simulink model "Simulation"  (R2024b)
settings: Solver=VariableStepAuto  StartTime=0.0  StopTime=10  RelTol=1e-3
model workspace (MAT data in the model file):
  PowerToForce = 0.0001
settings Model: Creator=fears  LastModifiedBy=fears

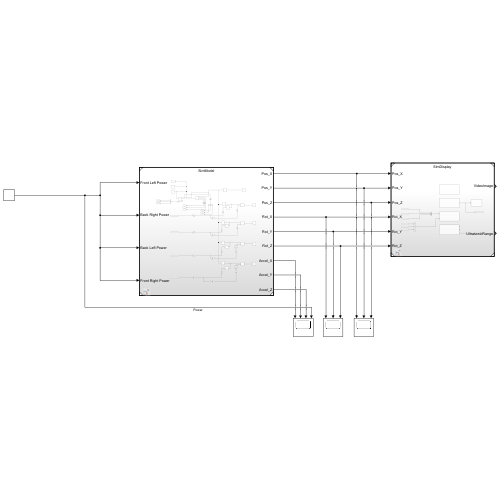
[thumbnail: Simulink's stored preview of the top-level diagram]
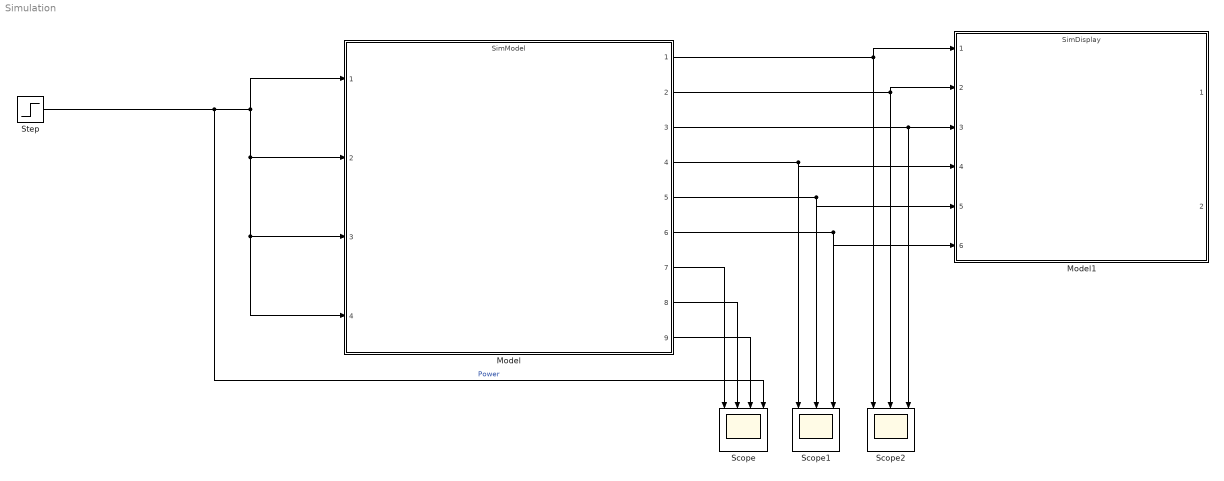
== system Simulation ==
  Model : ModelReference  ModelNameDialog=SimModel.slx  SimulationMode=Normal  ModelReferenceVersion=1.70
  Model1 : ModelReference  ModelNameDialog=SimDisplay.slx  SimulationMode=Normal  ModelReferenceVersion=1.24
  Scope : Scope  NumInputPorts=4
  Scope1 : Scope  NumInputPorts=3
  Scope2 : Scope  NumInputPorts=3
  Step : Step  SampleTime=0
  wires:
  Step/1 -> Scope/4, Model/1, Model/3, Model/4, Model/2  "Power"
  Model/1 -> Scope2/1, Model1/1
  Model/2 -> Model1/2, Scope2/2
  Model/3 -> Model1/3, Scope2/3
  Model/4 -> Scope1/1, Model1/4
  Model/5 -> Model1/5, Scope1/2
  Model/6 -> Model1/6, Scope1/3
  Model/7 -> Scope/1
  Model/8 -> Scope/2
  Model/9 -> Scope/3
